simulink model "assignment1_alt"  (R2020a)
settings: Solver=FixedStepAuto  StartTime=0.0  StopTime=5  FixedStep=1e-3  RelTol=1e-3  EnableMultiTasking=on
model workspace (MAT data in the model file):
  ATR_CMP_REF_PWM_PERCENTAGE = 50
  PACING_REF_PWM_DUTY_PERCENTAGE = 50
  VENT_CMP_REF_PWM_PERCENTAGE = 50
libraries: frdmk64flib x1
settings Model: ExtModeTrigDuration=5  OrderedModelArguments=off  Creator=John  LastModifiedBy=zhanz173
settings OptimizationCC: EnhancedBackFolding=on  PassReuseOutputArgsAs=Individual arguments  ZeroExternalMemoryAtStartup=off  ZeroInternalMemoryAtStartup=off  MaxStackSize=64  OptimizeBlockOrder=speed  DifferentSizesBufferReuse=on  OptimizationCustomize=off  EfficientTunableParamExpr=on
settings DebuggingCC: ParameterTunabilityLossMsg=error
settings HardwareCC: ProdBitPerPointer=32  ProdBitPerSizeT=32  ProdBitPerPtrDiffT=32  ProdLargestAtomicInteger=Long  ProdLargestAtomicFloat=Double  ProdWordSize=32  ProdHWDeviceType=ARM Compatible->ARM Cortex
settings SFSimCC: MATLABDynamicMemAlloc=off
settings RTWCC: SystemTargetFile=ert.tlc  HardwareBoard=NXP FRDM-K64F  TemplateMakefile=ert_default_tmf  Toolchain=GNU Tools for ARM Embedded Processors
settings CodeAppCC: ForceParamTrailComments=on  IgnoreCustomStorageClasses=off  OperatorAnnotations=on  SimulinkDataObjDesc=on  SFDataObjDesc=on  InsertBlockDesc=on

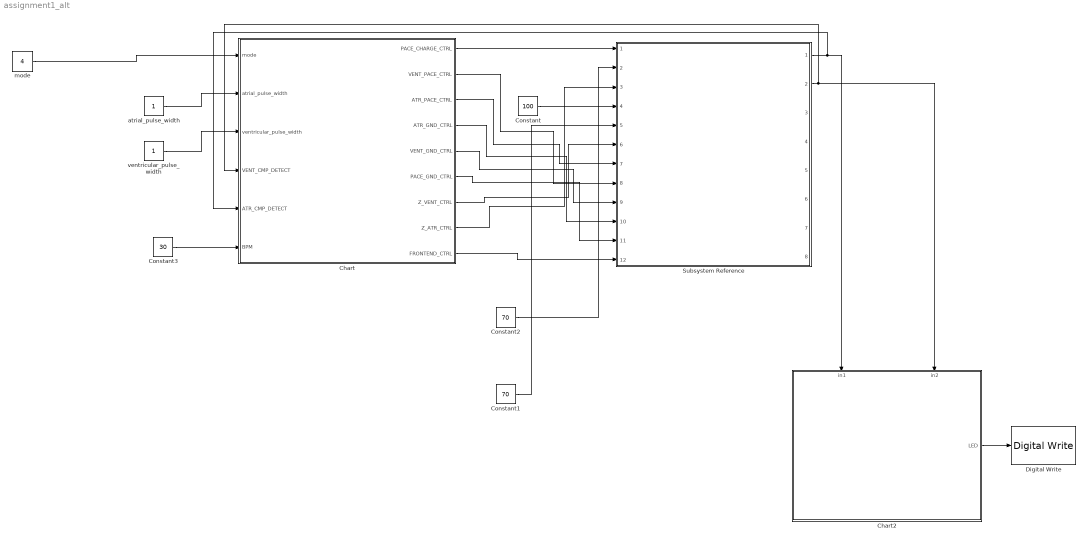
== system assignment1_alt ==
  Chart : Stateflow chart  TreatAsAtomicUnit=on
  Chart2 : Stateflow chart  TreatAsAtomicUnit=on
      settings: PortSchema="{\"entries\":[{\"content\":{\"sides\":[{\"content\":{\"connectorIds\":[]},\"type\":\"ConnectorPlacement.EquallySpacedRectSide\",\"uuid\":\"479640eb-eaca-44d1-8a3c-ce1ef181d33c\"},{\"content\":{\"connectorIds\":[\"Out1\"],\"side\":\"RIGHT\"},\"type\":\"ConnectorPlacement.EquallySpacedRectSide\",\"uuid\":\"1157b40f-c6cd-45ea-80e8-5724e4fde2e3\"},{\"content\":{\"connectorIds\":[\"In1\",\"In2\"],\"side\":\"TOP\"},\"type\":\"ConnectorPlacement.EquallySpacedRectSide\",\"uuid\":\"7c93b3c9-fbcd-45ae-8653-360703d4bd24\"}]},\"type\":\"ConnectorPlacement.EquallySpacedConnector\",\"uuid\":\"696d045e-2a8c-4d15-84cc-2302f7e6f390\"}],\"packageUris\":[\"http://schema.mathworks.com/mf0/Connector/19700101\"],\"version\":\"1.0\"}"
  Constant : Constant  Value=100
  Constant1 : Constant  Value=70
  Constant2 : Constant  Value=70
  Constant3 : Constant  Value=30
  Digital Write : frdmk64flib/Digital Write  Whichpin=RED_LED
  Subsystem Reference : Subsystem  ReferencedSubsystem=k64f_subsystem
  atrial_pulse_width : Constant
  mode : Constant  Value=4
  ventricular_pulse_width : Constant
  wires:
  mode/1 -> Chart/1(mode)
  Constant/1 -> Subsystem Reference/4
  atrial_pulse_width/1 -> Chart/2(atrial_pulse_width)
  ventricular_pulse_width/1 -> Chart/3(ventricular_pulse_width)
  Chart/8(Z_ATR_CTRL) -> Subsystem Reference/3
  Chart/7(Z_VENT_CTRL) -> Subsystem Reference/6
  Chart/4(ATR_GND_CTRL) -> Subsystem Reference/10
  Chart/3(ATR_PACE_CTRL) -> Subsystem Reference/7
  Chart/5(VENT_GND_CTRL) -> Subsystem Reference/9
  Chart/2(VENT_PACE_CTRL) -> Subsystem Reference/8
  Chart/1(PACE_CHARGE_CTRL) -> Subsystem Reference/1
  Chart/6(PACE_GND_CTRL) -> Subsystem Reference/11
  Subsystem Reference/1 -> Chart/5(ATR_CMP_DETECT), Chart2/1(in1)
  Constant2/1 -> Subsystem Reference/2
  Constant1/1 -> Subsystem Reference/5
  Chart/9(FRONTEND_CTRL) -> Subsystem Reference/12
  Subsystem Reference/2 -> Chart2/2(in2), Chart/4(VENT_CMP_DETECT)
  Chart2/1(LED) -> Digital Write/1
  Constant3/1 -> Chart/6(BPM)

== stateflow chart assignment1_alt/Chart2 ==
  state state1
    LED = 0;
  state delay2
  state state2
    LED = 1;
  state delay
    LED = 0;
  (default) -> state1
  delay2 -> state1 : after(500,msec)
  delay -> delay2 : [in1 == 1 || in2 == 1]
  state1 -> state2 : [in1 == 0 || in2 == 0]
  state2 -> delay : after(100,msec)
  data: in1 input; LED output; in2 input

== stateflow chart assignment1_alt/Chart ==
  state CHARGING
    entry:
    PACE_CHARGE_CTRL = 1;
    ATR_PACE_CTRL = 0;
    VENT_PACE_CTRL = 0;
    FRONTEND_CTRL = 0;
  state delay
  state Select_mode
    entry:
  state Atrial_Pacing
    entry:
    ATR_GND_CTRL = 0;
    VENT_GND_CTRL = 0;
    ATR_GND_CTRL = 0;
    PACE_CHARGE_CTRL = 0;
    ATR_PACE_CTRL = 1;
    VENT_PACE_CTRL = 0;
    PACE_GND_CTRL = 1;
  state No_Pacing
    entry:
    ATR_PACE_CTRL = 0;
    VENT_PACE_CTRL = 0;
  state Ventricular_Pacing
    entry:
    VENT_GND_CTRL = 0;
    ATR_GND_CTRL = 0;
    PACE_CHARGE_CTRL = 0;
    ATR_PACE_CTRL = 0;
    VENT_PACE_CTRL = 1;
    PACE_GND_CTRL = 1;
    Z_VENT_CTRL = 0;
    Z_ATR_CTRL = 0;
  state AAI
    entry:
    FRONTEND_CTRL = 1;
  state VVI
    entry:
    FRONTEND_CTRL = 1;
  state VAA_discharge
    entry:
    VENT_GND_CTRL = 0;
    ATR_GND_CTRL = 1;
    PACE_GND_CTRL = 1;
    ATR_PACE_CTRL = 0;
    VENT_PACE_CTRL = 0;
    Z_VENT_CTRL =0;
    Z_ATR_CTRL = 0;
  state Discharging
    entry:
    VENT_GND_CTRL = 1;
    ATR_GND_CTRL = 0;
    PACE_GND_CTRL = 1;
    ATR_PACE_CTRL = 0;
    VENT_PACE_CTRL = 0;
    Z_VENT_CTRL =0;
    Z_ATR_CTRL = 0;
  (default) -> CHARGING
  CHARGING -> delay [order 2] : [mode == 3 || mode == 4]
  VAA_discharge -> CHARGING
  No_Pacing -> CHARGING
  Discharging -> CHARGING
  CHARGING -> Select_mode [order 1] : after(60/BPM,sec)
  delay -> VVI [order 1] : [mode == 4]
  delay -> AAI [order 2] : [mode == 3]
  Select_mode -> Atrial_Pacing [order 3] : [mode == 1]
  Select_mode -> Ventricular_Pacing [order 1] : [mode == 2]
  Select_mode -> No_Pacing [order 2] : [mode == 5]
  AAI -> AAI [order 1] : [ATR_CMP_DETECT == 1]
  VVI -> VVI [order 1] : [VENT_CMP_DETECT == 1]
  AAI -> Atrial_Pacing [order 2] : after(60/BPM,sec)
  VVI -> Ventricular_Pacing [order 2] : after(60/BPM,sec)
  Ventricular_Pacing -> Discharging : after(ventricular_pulse_width,msec)
  Atrial_Pacing -> VAA_discharge : after(atrial_pulse_width,msec)
  data: PACE_CHARGE_CTRL output; VENT_PACE_CTRL output; ATR_PACE_CTRL output; ATR_GND_CTRL output; VENT_GND_CTRL output; PACE_GND_CTRL output; mode input; Z_VENT_CTRL output; Z_ATR_CTRL output; atrial_pulse_width input; ventricular_pulse_width input; VENT_CMP_DETECT input; ATR_CMP_DETECT input; FRONTEND_CTRL output; BPM input
